simulink model "SpeedHarm"  (Simulink 8.2)
settings: Solver=ode1  StartTime=0.0  StopTime=Inf  FixedStep=0.001  RelTol=1e-3
PostLoadFcn:
  | , if any(exist('dsrtsu_mdlpostloadfcn', 'file') == [2, 3, 6]), try dsrtsu_mdlpostloadfcn('Execute', bdroot); catch fprintf('Error in PostLoadFcn (dsrtsu_mdlpostloadfcn) for model "%s":\n %s\n', bdroot, lasterr); end, end,
undefined symbols (not defined in the file): AccelCommandMode, AutoStateEnum, command_mode, max_accel_m_s2, override_enabled, speed_command_m_s, wrench_effort_command
libraries: simulink x33, carma_platform x3, srx_platform x3, dsrc_transmitter x2, rtiethernetudplib x2, rtitttasklib x2, parse_utils x1, rtican x1
(part 2 of 2)

== system SpeedHarm/Write CACC Data/Veh 3 Data Write ==
  DSRC Bus : Inport
  Action Port : ActionPort  ActionType=case
  Bus Selector : BusSelector  OutputSignals=signal1,signal2,signal3,signal4,signal5,signal6,signal7,signal8,signal9,signal10,signal11,signal12,signal13,signal14,signal15,signal16,signal17,signal18,signal19,signal20,signal21,signal22,signal23,signal24,signal25,signal26
  Data Store Write : DataStoreWrite  DataStoreName=BSMStoreSignal  DataStoreElements=BSMStoreSignal.Veh3BSM.grpID#BSMStoreSignal.Veh3BSM.grpSize#BSMStoreSignal.Veh3BSM.grpMode#BSMStoreSignal.Veh3BSM.grpManDes#BSMStoreSignal.Veh3BSM.grpManID#BSMStoreSignal.Veh3BSM.vehID#BSMStoreSignal.Veh3BSM.frntCutIn#BSMStoreSignal.Veh3BSM.vehGrpPos#BSMStoreSignal.Veh3BSM.vehFltMode#BSMStoreSignal.Veh3BSM.vehManDes#BSMStoreSignal.Veh3BSM.vehManID#BSMStoreSignal.Veh3BSM.distToPVeh_m#BSMStoreSignal.Veh3BSM.relSpdPVeh_m_s#BSMStoreSignal.Veh3BSM.distToLVeh_m#BSMStoreSignal.Veh3BSM.relSpdLVeh_m_s#BSMStoreSignal.Veh3BSM.desTGapPVeh_s#BSMStoreSignal.Veh3BSM.desTGapLVeh_s#BSMStoreSignal.Veh3BSM.estDisPVeh_m#BSMStoreSignal.Veh3BSM.estDisLVeh_m#BSMStoreSignal.Veh3BSM.desSpeed_m_s#BSMStoreSignal.Veh3BSM.desTrq_N_m#BSMStoreSignal.Veh3BSM.userDE1#BSMStoreSignal.Veh3BSM.userDE2#BSMStoreSignal.Veh3BSM.userDE3#BSMStoreSignal.Veh3BSM.userDE4#BSMStoreSignal.Veh3BSM.userDE5
  wires:
  Bus Selector/26 -> Data Store Write/26  "<signal26>"
  Bus Selector/25 -> Data Store Write/25  "<signal25>"
  Bus Selector/24 -> Data Store Write/24  "<signal24>"
  Bus Selector/23 -> Data Store Write/23  "<signal23>"
  Bus Selector/22 -> Data Store Write/22  "<signal22>"
  Bus Selector/21 -> Data Store Write/21  "<signal21>"
  Bus Selector/20 -> Data Store Write/20  "<signal20>"
  Bus Selector/19 -> Data Store Write/19  "<signal19>"
  Bus Selector/18 -> Data Store Write/18  "<signal18>"
  Bus Selector/17 -> Data Store Write/17  "<signal17>"
  Bus Selector/16 -> Data Store Write/16  "<signal16>"
  Bus Selector/15 -> Data Store Write/15  "<signal15>"
  Bus Selector/14 -> Data Store Write/14  "<signal14>"
  Bus Selector/13 -> Data Store Write/13  "<signal13>"
  Bus Selector/12 -> Data Store Write/12  "<signal12>"
  Bus Selector/11 -> Data Store Write/11  "<signal11>"
  Bus Selector/10 -> Data Store Write/10  "<signal10>"
  Bus Selector/9 -> Data Store Write/9  "<signal9>"
  Bus Selector/8 -> Data Store Write/8  "<signal8>"
  Bus Selector/7 -> Data Store Write/7  "<signal7>"
  Bus Selector/6 -> Data Store Write/6  "<signal6>"
  Bus Selector/5 -> Data Store Write/5  "<signal5>"
  Bus Selector/4 -> Data Store Write/4  "<signal4>"
  Bus Selector/3 -> Data Store Write/3  "<signal3>"
  Bus Selector/2 -> Data Store Write/2  "<signal2>"
  Bus Selector/1 -> Data Store Write/1  "<signal1>"
  DSRC Bus/1 -> Bus Selector/1

== system SpeedHarm/Write CACC Data/Veh 4 Data Write ==
  DSRC Bus : Inport
  Action Port : ActionPort  ActionType=case
  Bus Selector : BusSelector  OutputSignals=signal1,signal2,signal3,signal4,signal5,signal6,signal7,signal8,signal9,signal10,signal11,signal12,signal13,signal14,signal15,signal16,signal17,signal18,signal19,signal20,signal21,signal22,signal23,signal24,signal25,signal26
  Data Store Write : DataStoreWrite  DataStoreName=BSMStoreSignal  DataStoreElements=BSMStoreSignal.Veh4BSM.grpID#BSMStoreSignal.Veh4BSM.grpSize#BSMStoreSignal.Veh4BSM.grpMode#BSMStoreSignal.Veh4BSM.grpManDes#BSMStoreSignal.Veh4BSM.grpManID#BSMStoreSignal.Veh4BSM.vehID#BSMStoreSignal.Veh4BSM.frntCutIn#BSMStoreSignal.Veh4BSM.vehGrpPos#BSMStoreSignal.Veh4BSM.vehFltMode#BSMStoreSignal.Veh4BSM.vehManDes#BSMStoreSignal.Veh4BSM.vehManID#BSMStoreSignal.Veh4BSM.distToPVeh_m#BSMStoreSignal.Veh4BSM.relSpdPVeh_m_s#BSMStoreSignal.Veh4BSM.distToLVeh_m#BSMStoreSignal.Veh4BSM.relSpdLVeh_m_s#BSMStoreSignal.Veh4BSM.desTGapPVeh_s#BSMStoreSignal.Veh4BSM.desTGapLVeh_s#BSMStoreSignal.Veh4BSM.estDisPVeh_m#BSMStoreSignal.Veh4BSM.estDisLVeh_m#BSMStoreSignal.Veh4BSM.desSpeed_m_s#BSMStoreSignal.Veh4BSM.desTrq_N_m#BSMStoreSignal.Veh4BSM.userDE1#BSMStoreSignal.Veh4BSM.userDE2#BSMStoreSignal.Veh4BSM.userDE3#BSMStoreSignal.Veh4BSM.userDE4#BSMStoreSignal.Veh4BSM.userDE5
  wires:
  Bus Selector/26 -> Data Store Write/26  "<signal26>"
  Bus Selector/25 -> Data Store Write/25  "<signal25>"
  Bus Selector/24 -> Data Store Write/24  "<signal24>"
  Bus Selector/23 -> Data Store Write/23  "<signal23>"
  Bus Selector/22 -> Data Store Write/22  "<signal22>"
  Bus Selector/21 -> Data Store Write/21  "<signal21>"
  Bus Selector/20 -> Data Store Write/20  "<signal20>"
  Bus Selector/19 -> Data Store Write/19  "<signal19>"
  Bus Selector/18 -> Data Store Write/18  "<signal18>"
  Bus Selector/17 -> Data Store Write/17  "<signal17>"
  Bus Selector/16 -> Data Store Write/16  "<signal16>"
  Bus Selector/15 -> Data Store Write/15  "<signal15>"
  Bus Selector/14 -> Data Store Write/14  "<signal14>"
  Bus Selector/13 -> Data Store Write/13  "<signal13>"
  Bus Selector/12 -> Data Store Write/12  "<signal12>"
  Bus Selector/11 -> Data Store Write/11  "<signal11>"
  Bus Selector/10 -> Data Store Write/10  "<signal10>"
  Bus Selector/9 -> Data Store Write/9  "<signal9>"
  Bus Selector/8 -> Data Store Write/8  "<signal8>"
  Bus Selector/7 -> Data Store Write/7  "<signal7>"
  Bus Selector/6 -> Data Store Write/6  "<signal6>"
  Bus Selector/5 -> Data Store Write/5  "<signal5>"
  Bus Selector/4 -> Data Store Write/4  "<signal4>"
  Bus Selector/3 -> Data Store Write/3  "<signal3>"
  Bus Selector/2 -> Data Store Write/2  "<signal2>"
  Bus Selector/1 -> Data Store Write/1  "<signal1>"
  DSRC Bus/1 -> Bus Selector/1

== system SpeedHarm/Write CACC Data/Veh 5 Data Write ==
  DSRC Bus : Inport
  Action Port : ActionPort  ActionType=case
  Bus Selector : BusSelector  OutputSignals=signal1,signal2,signal3,signal4,signal5,signal6,signal7,signal8,signal9,signal10,signal11,signal12,signal13,signal14,signal15,signal16,signal17,signal18,signal19,signal20,signal21,signal22,signal23,signal24,signal25,signal26
  Data Store Write : DataStoreWrite  DataStoreName=BSMStoreSignal  DataStoreElements=BSMStoreSignal.Veh5BSM.grpID#BSMStoreSignal.Veh5BSM.grpSize#BSMStoreSignal.Veh5BSM.grpMode#BSMStoreSignal.Veh5BSM.grpManDes#BSMStoreSignal.Veh5BSM.grpManID#BSMStoreSignal.Veh5BSM.vehID#BSMStoreSignal.Veh5BSM.frntCutIn#BSMStoreSignal.Veh5BSM.vehGrpPos#BSMStoreSignal.Veh5BSM.vehFltMode#BSMStoreSignal.Veh5BSM.vehManDes#BSMStoreSignal.Veh5BSM.vehManID#BSMStoreSignal.Veh5BSM.distToPVeh_m#BSMStoreSignal.Veh5BSM.relSpdPVeh_m_s#BSMStoreSignal.Veh5BSM.distToLVeh_m#BSMStoreSignal.Veh5BSM.relSpdLVeh_m_s#BSMStoreSignal.Veh5BSM.desTGapPVeh_s#BSMStoreSignal.Veh5BSM.desTGapLVeh_s#BSMStoreSignal.Veh5BSM.estDisPVeh_m#BSMStoreSignal.Veh5BSM.estDisLVeh_m#BSMStoreSignal.Veh5BSM.desSpeed_m_s#BSMStoreSignal.Veh5BSM.desTrq_N_m#BSMStoreSignal.Veh5BSM.userDE1#BSMStoreSignal.Veh5BSM.userDE2#BSMStoreSignal.Veh5BSM.userDE3#BSMStoreSignal.Veh5BSM.userDE4#BSMStoreSignal.Veh5BSM.userDE5
  wires:
  Bus Selector/26 -> Data Store Write/26  "<signal26>"
  Bus Selector/25 -> Data Store Write/25  "<signal25>"
  Bus Selector/24 -> Data Store Write/24  "<signal24>"
  Bus Selector/23 -> Data Store Write/23  "<signal23>"
  Bus Selector/22 -> Data Store Write/22  "<signal22>"
  Bus Selector/21 -> Data Store Write/21  "<signal21>"
  Bus Selector/20 -> Data Store Write/20  "<signal20>"
  Bus Selector/19 -> Data Store Write/19  "<signal19>"
  Bus Selector/18 -> Data Store Write/18  "<signal18>"
  Bus Selector/17 -> Data Store Write/17  "<signal17>"
  Bus Selector/16 -> Data Store Write/16  "<signal16>"
  Bus Selector/15 -> Data Store Write/15  "<signal15>"
  Bus Selector/14 -> Data Store Write/14  "<signal14>"
  Bus Selector/13 -> Data Store Write/13  "<signal13>"
  Bus Selector/12 -> Data Store Write/12  "<signal12>"
  Bus Selector/11 -> Data Store Write/11  "<signal11>"
  Bus Selector/10 -> Data Store Write/10  "<signal10>"
  Bus Selector/9 -> Data Store Write/9  "<signal9>"
  Bus Selector/8 -> Data Store Write/8  "<signal8>"
  Bus Selector/7 -> Data Store Write/7  "<signal7>"
  Bus Selector/6 -> Data Store Write/6  "<signal6>"
  Bus Selector/5 -> Data Store Write/5  "<signal5>"
  Bus Selector/4 -> Data Store Write/4  "<signal4>"
  Bus Selector/3 -> Data Store Write/3  "<signal3>"
  Bus Selector/2 -> Data Store Write/2  "<signal2>"
  Bus Selector/1 -> Data Store Write/1  "<signal1>"
  DSRC Bus/1 -> Bus Selector/1

== system SpeedHarm/Write CACC Data/Vehicle Identification Error ==
  note: Error Handling Goes Here
  Action Port : ActionPort  ActionType=default

== system SpeedHarm/Write CACC Data/Vehicle Identification Error1 ==
  note: Error Handling Goes Here
  Action Port : ActionPort  ActionType=case

== system SpeedHarm/RTI Data/RTI Data Store/RTI Data Store ==
  RTI Data Store : Subsystem  mask(RTI_DATA_STORE){}
      mask help:
      | RTI Data Store Block. This block is used by RTI to store internal model dependent data. Deleting this block will result in data loss.
      |
      | NEVER DELETE, COPY, OR MODIFY THIS BLOCK!
      mask Help:
      | RTI Data Store Block. This block is used by RTI to store internal model dependent data. Deleting this block will result in data loss.
      | 
      | NEVER DELETE, COPY, OR MODIFY THIS BLOCK!
      mask Display: text(0.5, 0.5, ' ', 'HorizontalAlignment', 'center');

== system SpeedHarm/Speed Harm Control Code/Radar Validation/Object in path ==
  lat pos [m] : Inport
  steering angle [deg] : Inport  Port=2
  Abs : Abs
  DocBlock : simulink/Model-Wide Utilities/DocBlock  DocumentType=Text
  Half Lane Width [m] : Constant  Value=2
  Relational Operator : RelationalOperator  Operator=<=  OutDataTypeStr=boolean
  in path : Outport
  wires:
  lat pos [m]/1 -> Abs/1
  Half Lane Width [m]/1 -> Relational Operator/2
  Relational Operator/1 -> in path/1
  Abs/1 -> Relational Operator/1

== system SpeedHarm/Speed Harm Control Code/SRX PC2 UDP Handler/SRX PC2 UDP RX Handler ==
  ETHERNET_UDP_RX_COMMAND : rtiethernetudplib/ETHERNET_UDP_RX_BL1  InterfaceName=rti_ethernet_interface_name  BoardType=ETH Type 1  ModuleNo=1  ChannelNo=1  SocketNo=4  MaxMessageSize=5  LocalSocket=192.168.88.21:5003  RemoteSocket=192.168.88.10:5003  DSProperties=struct('RTI',struct('Version',uint32(1),'BlockType',struct('isSLSource',uint8(1),'isSLSink',uint8(0),'isHWSource',uint8(0),'isHWSink',uint8(1),'isSetup',uint8(0),'isInline',uint8(1),'isNonInline',uint8(1),'isInterrupt',uint8(0),'isChannelwise',uint8(1)),'IOBoardType','DSETHERNETUDP','UnitType','ETHUDP','Identifier','RX','DialogType','SL','BlockSet','RTIETHERNETUDP','SlaveProcessor','NONE'))  RTIBlockInterface=struct('OutputPortsWidth',int32([1 1 1]),'OutputPortsActive',[1 1 1],'OutputPortsName',{{'Data',['Message Size'],'Status'}},'OutputPortsDataType',{{'SS_UINT32','SS_INT32','SS_BOOLEAN'}},'BlockDisplay',{{['Ethernet UDP Receive\nBoard Type: ETH Type 1\nModule: 1\nSocket: 4\nMaximum Message Size: 5'],'center'}},'IconTransparency','on','InitLevel',3,'BlockName',struct('Token',{{'ETHERNET_UDP_RX_BL1'}}),'MaskDescription',['To receive messages from the Ethernet UDP interface.'])  RTIBlockParameters=struct('InterfaceName',{{'rti_ethernet_interface_name','OFF',[]}},'BoardType',{{1,'OFF',[]}},'ModuleNo',{{1,'OFF',[1 16]}},'ChannelNo',{{1,'OFF',[1 2]}},'SocketNo',{{4,'OFF',[1 4]}},'MaxMessageSize',{{5,'ON',[1 1472]}},'LocalSocket',{{'192.168.88.21:5003','OFF',[]}},'RemoteSocket',{{'192.168.88.10:5003','OFF',[]}})  RTISFcnParameters=struct('InterfaceName','char','BoardType','double','ModuleNo','double','ChannelNo','double','SocketNo','double','MaxMessageSize','double','LocalSocket','char','RemoteSocket','char')  RTIBlockParaDefault=struct('InterfaceName','rti_ethernet_interface_name','BoardType',1,'ModuleNo',1,'ChannelNo',1,'SocketNo',1,'MaxMessageSize',625,'LocalSocket','XXX.XXX.XXX.XXX:5000','RemoteSocket','XXX.XXX.XXX.XXX:5000')
  UDP RX Data : Outport
  cmd_msg_size : Outport  Port=2
  cmd_msg_status : Outport  Port=3
  wires:
  ETHERNET_UDP_RX_COMMAND/1 -> UDP RX Data/1  "Data from PC2"
  ETHERNET_UDP_RX_COMMAND/2 -> cmd_msg_size/1
  ETHERNET_UDP_RX_COMMAND/3 -> cmd_msg_status/1

== system SpeedHarm/Speed Harm Control Code/SRX PC2 UDP Handler/SRX PC2 UDP TX Handler ==
  UDP TX data : Inport
  msg size (bytes) : Inport  Port=2
  Constant1 : Constant  OutDataTypeStr=boolean
  ETHERNET_UDP_TX_BL1 : rtiethernetudplib/ETHERNET_UDP_TX_BL1  InterfaceName=rti_ethernet_interface_name  BoardType=ETH Type 1  ModuleNo=1  ChannelNo=1  SocketNo=4  MaxMessageSize=20  SendTimeout=0.01  LocalSocket=192.168.88.21:5003  RemoteSocket=192.168.88.10:5003  DSProperties=struct('RTI',struct('Version',uint32(2),'BlockType',struct('isSLSource',uint8(1),'isSLSink',uint8(1),'isHWSource',uint8(1),'isHWSink',uint8(1),'isSetup',uint8(0),'isInline',uint8(1),'isNonInline',uint8(1),'isInterrupt',uint8(0),'isChannelwise',uint8(1)),'IOBoardType','DSETHERNETUDP','UnitType','ETHUDP','Identifier','TX','DialogType','SL','BlockSet','RTIETHERNETUDP','SlaveProcessor','NONE'))  RTIBlockInterface=struct('OutputPortsWidth',int32(1),'OutputPortsActive',1,'OutputPortsName',{{'Status'}},'OutputPortsDataType',{{'SS_UINT16'}},'InputPortsWidth',int32([1 1 1]),'InputPortsActive',[1 1 1],'InputPortsName',{{'Data',['Message Size'],'Enable'}},'InputPortsDataType',{{'SS_UINT32','SS_INT32','SS_BOOLEAN'}},'BlockDisplay',{{['Ethernet UDP Transmit\nBoard Type: ETH Type 1\nModule: 1\nSocket: 4\nMaximum Message Size: 20'],'center'}},'IconTransparency','on','InitLevel',3,'BlockName',struct('Token',{{'ETHERNET_UDP_TX_BL1'}}),'MaskDescription',['To send messages via the Ethernet UDP interface.'])  RTIBlockParameters=struct('InterfaceName',{{'rti_ethernet_interface_name','OFF',[]}},'BoardType',{{1,'OFF',[]}},'ModuleNo',{{1,'OFF',[1 16]}},'ChannelNo',{{1,'OFF',[1 2]}},'SocketNo',{{4,'OFF',[1 4]}},'MaxMessageSize',{{20,'ON',[1 1472]}},'SendTimeout',{{0.01,'ON',[1e-05 2]}},'LocalSocket',{{'192.168.88.21:5003','OFF',[]}},'RemoteSocket',{{'192.168.88.10:5003','OFF',[]}})  RTISFcnParameters=struct('InterfaceName','char','BoardType','double','ModuleNo','double','ChannelNo','double','SocketNo','double','MaxMessageSize','double','SendTimeout','double','LocalSocket','char','RemoteSocket','char')  RTIBlockParaDefault=struct('InterfaceName','rti_ethernet_interface_name','BoardType',1,'ModuleNo',1,'ChannelNo',1,'SocketNo',1,'MaxMessageSize',625,'SendTimeout',0.0005,'LocalSocket','XXX.XXX.XXX.XXX:5000','RemoteSocket','XXX.XXX.XXX.XXX:5000')
  Status : Outport
  wires:
  UDP TX data/1 -> ETHERNET_UDP_TX_BL1/1  "Data to PC2"
  msg size (bytes)/1 -> ETHERNET_UDP_TX_BL1/2
  Constant1/1 -> ETHERNET_UDP_TX_BL1/3
  ETHERNET_UDP_TX_BL1/1 -> Status/1

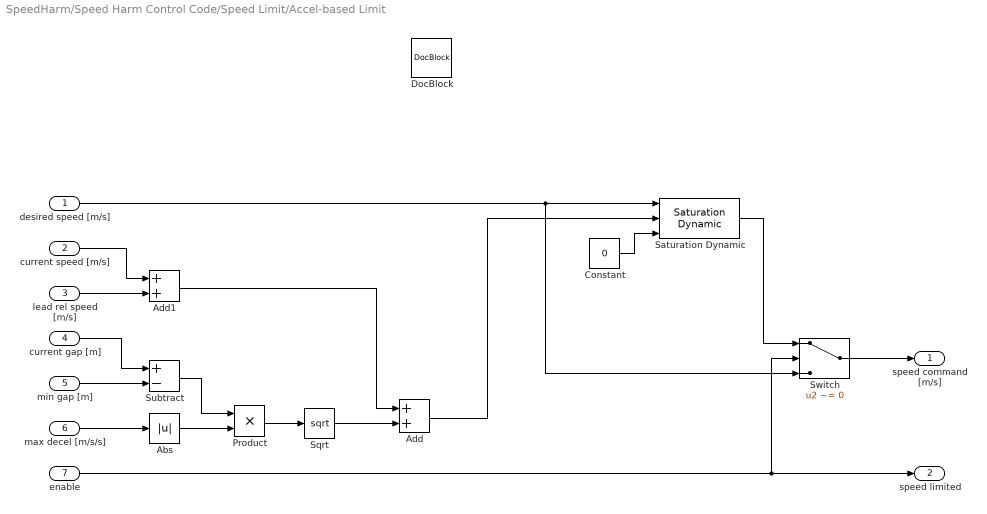
== system SpeedHarm/Speed Harm Control Code/Speed Limit/Accel-based Limit ==
  desired speed [m/s] : Inport
  current speed [m/s] : Inport  Port=2
  lead rel speed [m/s] : Inport  Port=3
  current gap [m] : Inport  Port=4
  min gap [m] : Inport  Port=5
  max decel [m/s/s] : Inport  Port=6
  enable : Inport  Port=7
  Abs : Abs
  Add : Sum
  Add1 : Sum
  Constant : Constant  Value=0
  DocBlock : simulink/Model-Wide Utilities/DocBlock  DocumentType=Text
  Product : Product
  Saturation Dynamic : simulink/Discontinuities/Saturation Dynamic  OutMin=[]  OutMax=[]  OutDataTypeStr=Inherit: Same as second input  OutDataType=fixdt(1, 16)  OutScaling=2^-10  DoSatur=off
  Sqrt : Sqrt  SaturateOnIntegerOverflow=on
  Subtract : Sum  Inputs=+-
  Switch : Switch  Criteria=u2 ~= 0
  speed command [m/s] : Outport
  speed limited : Outport  Port=2
  wires:
  enable/1 -> Switch/2, speed limited/1
  Saturation Dynamic/1 -> Switch/1
  Switch/1 -> speed command [m/s]/1
  Constant/1 -> Saturation Dynamic/3
  max decel [m/s/s]/1 -> Abs/1
  Subtract/1 -> Product/1
  Product/1 -> Sqrt/1
  Abs/1 -> Product/2
  current gap [m]/1 -> Subtract/1
  min gap [m]/1 -> Subtract/2
  desired speed [m/s]/1 -> Switch/3, Saturation Dynamic/1
  Sqrt/1 -> Add/2
  current speed [m/s]/1 -> Add1/1
  lead rel speed [m/s]/1 -> Add1/2
  Add1/1 -> Add/1
  Add/1 -> Saturation Dynamic/2

== system SpeedHarm/Speed Harm Control Code/Speed Limit/Check Auto Source ==
  current gap [m] : Inport
  min gap [m] : Inport  Port=2
  relative spd [m/s] : Inport  Port=3
  max decel [m/s/s] : Inport  Port=4
  Check Gap : Subsystem
  Check Speed Delta : Subsystem
  DocBlock : simulink/Model-Wide Utilities/DocBlock  DocumentType=Text
  Gap Warn : Outport
  Spd Warn : Outport  Port=2
  wires:
  relative spd [m/s]/1 -> Check Speed Delta/1(rel speed [m/s])
  max decel [m/s/s]/1 -> Check Speed Delta/3(max decel  [m/s/s])
  Check Speed Delta/1(speed warning) -> Spd Warn/1
  current gap [m]/1 -> Check Gap/1(current gap [m]), Check Speed Delta/2(current gap [m])
  min gap [m]/1 -> Check Gap/2(min gap [m])
  Check Gap/1(gap warning) -> Gap Warn/1

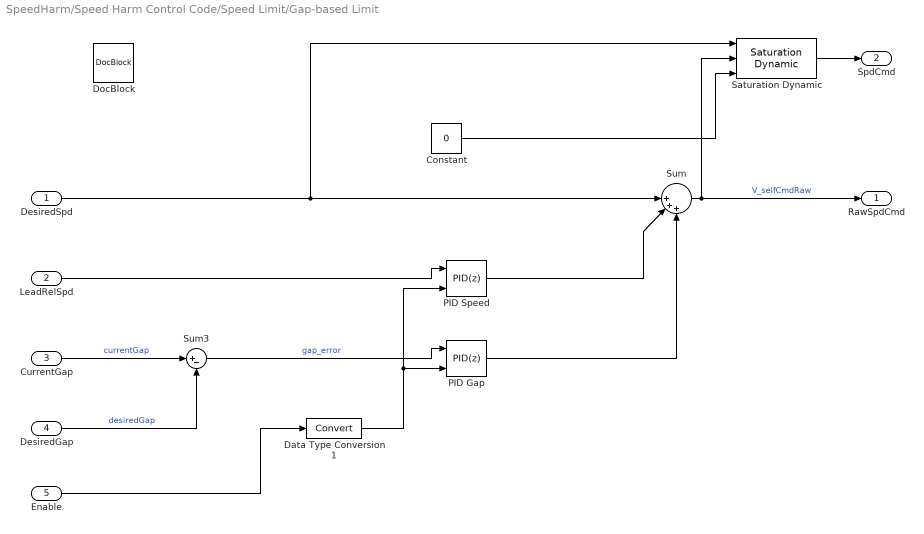
== system SpeedHarm/Speed Harm Control Code/Speed Limit/Gap-based Limit ==
  DesiredSpd : Inport
  LeadRelSpd : Inport  Port=2
  CurrentGap : Inport  Port=3
  DesiredGap : Inport  Port=4
  Enable : Inport  Port=5
  Constant : Constant  Value=0
  Data Type Conversion1 : DataTypeConversion
  DocBlock : simulink/Model-Wide Utilities/DocBlock  DocumentType=Text
      content=|
      | This block handles speed and gap control.
      |
      | This block attempts to minimize gap error via control of speed. It utilizes
      | a PID controller with gap error as the process variable and speed as the
      | manipulated variable. This PID outputs a speed command which is relative to
      | the lead vehicle's speed, thus it is added to the lead vehicle's speed to
      | get a desired speed value. Once the desired speed is computed it is run
      | through a saturation function to limit the values to between 0 and 1.2 *
      | Lead Vehicle Speed + 10.
  PID Gap : simulink/Continuous/PID Controller  Controller=PID  TimeDomain=Discrete-time  SampleTime=-1  IntegratorMethod=Forward Euler  FilterMethod=Forward Euler  Form=Parallel  P=0.5  I=0.01  D=0.1  N=10  InitialConditionSource=internal  InitialConditionForIntegrator=0  InitialConditionForFilter=0  ExternalReset=either  LimitOutput=on  UpperSaturationLimit=2  LowerSaturationLimit=-12  LinearizeAsGain=on  AntiWindupMode=back-calculation  Kb=1  TrackingMode=off  Kt=1  PParamMin=[]  PParamMax=[]  IParamMin=[]  IParamMax=[]  DParamMin=[]  DParamMax=[]  NParamMin=[]  NParamMax=[]  KbParamMin=[]  KbParamMax=[]  KtParamMin=[]  KtParamMax=[]  POutMin=[]  POutMax=[]  IOutMin=[]  IOutMax=[]  DOutMin=[]  DOutMax=[]  NOutMin=[]  NOutMax=[]  KbOutMin=[]  KbOutMax=[]  KtOutMin=[]  KtOutMax=[]  IntegratorOutMin=[]  IntegratorOutMax=[]  FilterOutMin=[]  FilterOutMax=[]  SumOutMin=[]  SumOutMax=[]  SumI1OutMin=[]  SumI1OutMax=[]  SumI2OutMin=[]  SumI2OutMax=[]  SumI3OutMin=[]  SumI3OutMax=[]  SumDOutMin=[]  SumDOutMax=[]  SaturationOutMin=[]  SaturationOutMax=[]  IntegratorContinuousStateAttributes=''  IntegratorStateMustResolveToSignalObject=off  IntegratorRTWStateStorageClass=Auto  FilterContinuousStateAttributes=''  FilterStateMustResolveToSignalObject=off  FilterRTWStateStorageClass=Auto
  PID Speed : simulink/Continuous/PID Controller  Controller=PID  TimeDomain=Discrete-time  SampleTime=-1  IntegratorMethod=Forward Euler  FilterMethod=Forward Euler  Form=Parallel  P=0.2  I=0  D=0  N=10  InitialConditionSource=internal  InitialConditionForIntegrator=0  InitialConditionForFilter=0  ExternalReset=either  LimitOutput=on  UpperSaturationLimit=2  LowerSaturationLimit=-12  LinearizeAsGain=on  AntiWindupMode=back-calculation  Kb=1  TrackingMode=off  Kt=1  PParamMin=[]  PParamMax=[]  IParamMin=[]  IParamMax=[]  DParamMin=[]  DParamMax=[]  NParamMin=[]  NParamMax=[]  KbParamMin=[]  KbParamMax=[]  KtParamMin=[]  KtParamMax=[]  POutMin=[]  POutMax=[]  IOutMin=[]  IOutMax=[]  DOutMin=[]  DOutMax=[]  NOutMin=[]  NOutMax=[]  KbOutMin=[]  KbOutMax=[]  KtOutMin=[]  KtOutMax=[]  IntegratorOutMin=[]  IntegratorOutMax=[]  FilterOutMin=[]  FilterOutMax=[]  SumOutMin=[]  SumOutMax=[]  SumI1OutMin=[]  SumI1OutMax=[]  SumI2OutMin=[]  SumI2OutMax=[]  SumI3OutMin=[]  SumI3OutMax=[]  SumDOutMin=[]  SumDOutMax=[]  SaturationOutMin=[]  SaturationOutMax=[]  IntegratorContinuousStateAttributes=''  IntegratorStateMustResolveToSignalObject=off  IntegratorRTWStateStorageClass=Auto  FilterContinuousStateAttributes=''  FilterStateMustResolveToSignalObject=off  FilterRTWStateStorageClass=Auto
  Saturation Dynamic : simulink/Discontinuities/Saturation Dynamic  OutMin=[]  OutMax=[]  OutDataTypeStr=Inherit: Same as second input  OutDataType=fixdt(1, 16)  OutScaling=2^-10  DoSatur=off
  Sum : Sum  Inputs=||+++
  Sum3 : Sum  Inputs=|+-
  RawSpdCmd : Outport
  SpdCmd : Outport  Port=2
  wires:
  DesiredGap/1 -> Sum3/2  "desiredGap"
  CurrentGap/1 -> Sum3/1  "currentGap"
  Sum/1 -> RawSpdCmd/1, Saturation Dynamic/2  "V_selfCmdRaw"
  Constant/1 -> Saturation Dynamic/3
  DesiredSpd/1 -> Saturation Dynamic/1, Sum/1
  Sum3/1 -> PID Gap/1  "gap_error"
  LeadRelSpd/1 -> PID Speed/1
  PID Gap/1 -> Sum/3
  Saturation Dynamic/1 -> SpdCmd/1
  PID Speed/1 -> Sum/2
  Enable/1 -> Data Type Conversion1/1
  Data Type Conversion1/1 -> PID Speed/2, PID Gap/2

== system SpeedHarm/RTI Data/RTI Data Store/RTI Data Store/RTI Data Store ==
  RTI Data Store : Subsystem  mask(RTI_DATA_STORE){}
      mask help:
      | RTI Data Store Block. This block is used by RTI to store internal model dependent data. Deleting this block will result in data loss.
      |
      | NEVER DELETE, COPY, OR MODIFY THIS BLOCK!
      mask Help:
      | RTI Data Store Block. This block is used by RTI to store internal model dependent data. Deleting this block will result in data loss.
      | 
      | NEVER DELETE, COPY, OR MODIFY THIS BLOCK!
      mask Display: text(0.5, 0.5, ' ', 'HorizontalAlignment', 'center');

== system SpeedHarm/Speed Harm Control Code/Speed Limit/Check Auto Source/Check Gap ==
  current gap [m] : Inport
  min gap [m] : Inport  Port=2
  Compare To Zero : simulink/Logic and Bit Operations/Compare To Zero  relop=<=  OutDataTypeStr=uint8
  Hys High : Constant  Value=1.5
  Hys Low : Constant  Value=1.25
  Memory : Memory  InheritSampleTime=on
  Product : Product
  Subtract : Sum  Inputs=+-
  Switch1 : Switch  Criteria=u2 ~= 0
  gap warning : Outport
  wires:
  Subtract/1 -> Compare To Zero/1
  min gap [m]/1 -> Product/1
  Product/1 -> Subtract/2
  Hys Low/1 -> Switch1/3
  Memory/1 -> Switch1/2
  Compare To Zero/1 -> gap warning/1, Memory/1
  Hys High/1 -> Switch1/1
  Switch1/1 -> Product/2
  current gap [m]/1 -> Subtract/1

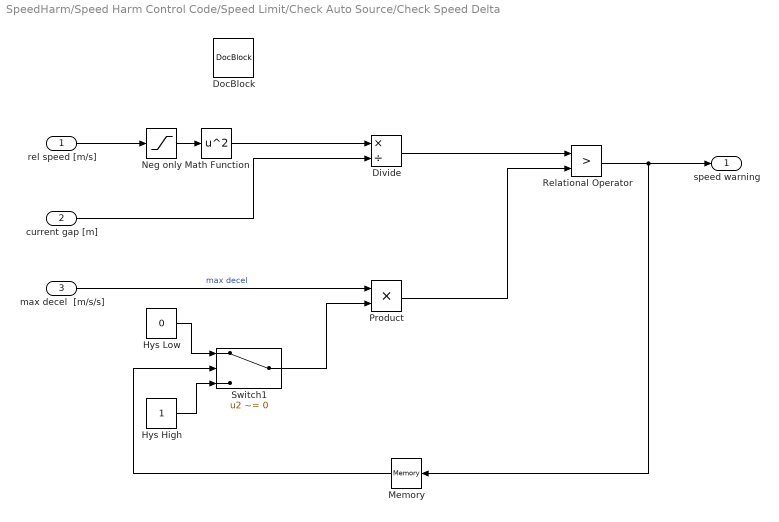
== system SpeedHarm/Speed Harm Control Code/Speed Limit/Check Auto Source/Check Speed Delta ==
  rel speed [m/s] : Inport
  current gap [m] : Inport  Port=2
  max decel  [m/s/s] : Inport  Port=3
  Divide : Product  Inputs=*/
  DocBlock : simulink/Model-Wide Utilities/DocBlock  DocumentType=Text
      content=|
      | This block checks that there is enough time to slow down to match a lead
      | vehicle's speed while staying below the max deceleration.
  Hys High : Constant
  Hys Low : Constant  Value=0
  Math Function : Math  Operator=square  SaturateOnIntegerOverflow=on
  Memory : Memory  InheritSampleTime=on
  Neg only : Saturate  UpperLimit=0  LowerLimit=-inf
  Product : Product
  Relational Operator : RelationalOperator  Operator=>  OutDataTypeStr='uint8'
  Switch1 : Switch  Criteria=u2 ~= 0
  speed warning : Outport
  wires:
  rel speed [m/s]/1 -> Neg only/1
  Math Function/1 -> Divide/1
  current gap [m]/1 -> Divide/2
  Divide/1 -> Relational Operator/1
  Switch1/1 -> Product/2
  Hys High/1 -> Switch1/3
  Memory/1 -> Switch1/2
  Relational Operator/1 -> Memory/1, speed warning/1
  Product/1 -> Relational Operator/2
  Hys Low/1 -> Switch1/1
  max decel  [m/s/s]/1 -> Product/1  "max decel"
  Neg only/1 -> Math Function/1

== system SpeedHarm/RTI Data/RTI Data Store/RTI Data Store/RTI Data Store/RTI Data Store ==

== matlab function Speed Harm Control Code/Lightbar Controller/MATLAB Function ==
  data: state input double; lightbar output double
function lightbar = lights(state)
%#codegen

lightbar = [false, false, false, false];

if state == MergeStateEnum.MERGE_REQUEST
    lightbar(2) = true;
end

if state == MergeStateEnum.F_MERGE_REQUEST_ACK
    lightbar(1) = true;
end

if state == MergeStateEnum.M_MERGE_READY || state == MergeStateEnum.F_MERGE_READY
    lightbar(2) = true;
    lightbar(1) = true;
end

if state == MergeStateEnum.M_MERGE_COMPLETE || state == MergeStateEnum.F_MERGE_COMPLETE
    lightbar(3) = true;
    lightbar(2) = true;
    lightbar(1) = true;
end
